simulink model "KR6_Decentralized_Trajectory"  (R2018a)
settings: Solver=VariableStepAuto  StartTime=0.0  StopTime=20  RelTol=1e-3
values from neighbouring files (symbols this model uses):
  Kd_Decent = zeros(7,7)    [ControlSetup.m]
  Kp_Decent = zeros(7,7)    [ControlSetup.m]
libraries: vrlib x8, KR6_Lib x2, dspinverses x1, realtime_pacer_lib x1
(part 1 of 2)
settings Model: Creator=Pedro Ramalho  LastModifiedBy=Pedro Ramalho
settings DataIOCC: ReturnWorkspaceOutputs=on  ReturnWorkspaceOutputsName=Centralized

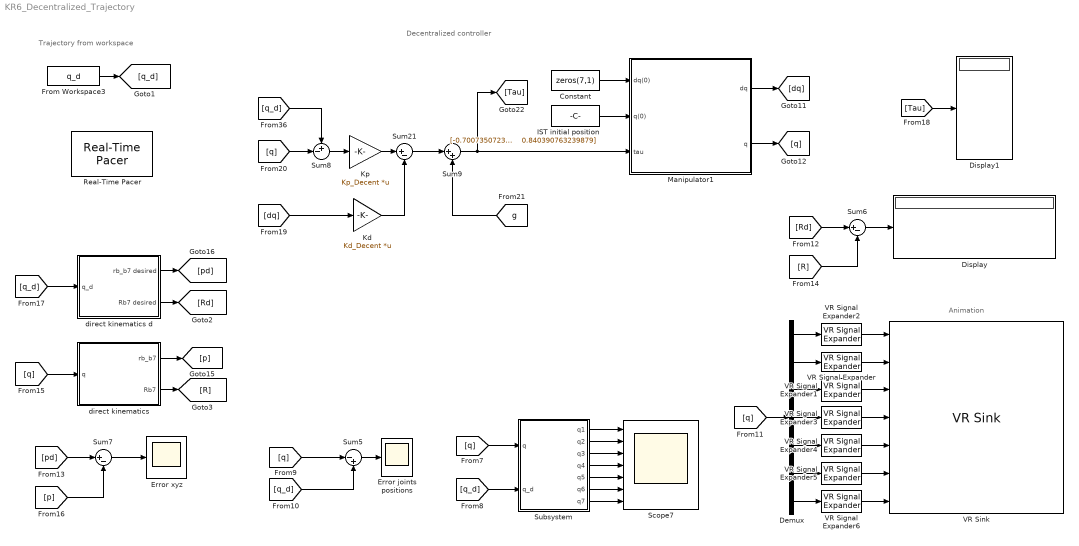
== system KR6_Decentralized_Trajectory ==
  note: Animation
  note: Trajectory from workspace
  note: Decentralized controller
  Constant : Constant  Value=zeros(7,1)
  Demux : Demux  Outputs=7
  Display : Display
  Display1 : Display
  Error joints positions : Scope
  Error xyz : Scope
  From Workspace3 : FromWorkspace  VariableName=q_d  SampleTime=0
  IST initial position : Constant  Value="[-0.700735072364346    0.260226322165590    -1.41409718169695    0.123044715609812    0.767247092108692    -0.379724450954367    0.840390763239879]"
  Kd : Gain  Gain=Kd_Decent  Multiplication=Matrix(K*u)
  Kp : Gain  Gain=Kp_Decent  Multiplication=Matrix(K*u)
  Manipulator1 : Subsystem
  Real-Time Pacer : realtime_pacer_lib/Real-Time Pacer  simTimePerRealTime=1
  Scope7 : Scope  NumInputPorts=7
  Subsystem : Subsystem
  Sum21 : Sum  Inputs=|+-
  Sum5 : Sum  Inputs=|-+
  Sum6 : Sum  Inputs=|+-
  Sum7 : Sum  Inputs=|+-
  Sum8 : Sum  Inputs=+-|
  Sum9 : Sum  Inputs=|++
  VR Signal Expander{,1,3..6} (6 alike) : vrlib/VR Signal Expander  outwidth=4  outidx=4
      settings: SourceProductName=Simulink 3D Animation  SourceProductBaseCode=VR
  VR Signal Expander2 : vrlib/VR Signal Expander  outwidth=3  outidx=3
      settings: SourceProductName=Simulink 3D Animation  SourceProductBaseCode=VR
  VR Sink : vrlib/VR Sink  InstantiateOnLoad=on  SampleTime=0.1  ViewEnable=on  RemoteChange=off  RemoteView=off  FieldsWritten=Jt1_DH_dv.translation.3.1.1.double#Jt2_DH_dv.rotation.4.1.1.double#Jt3_DH_dv.rotation.4.1.1.double#Jt4_DH_dv.rotation.4.1.1.double#Jt5_DH_dv.rotation.4.1.1.double#Jt6_DH_dv.rotation.4.1.1.double#Jt7_DH_dv.rotation.4.1.1.double  WorldFileName=vrrobotKR6.wrl  WorldDescription=D-H Reference Frames for Virtual Reality Robot  AutoView=off  VideoDimensions=[]  AllowVariableSize=off
      settings: SourceProductBaseCode=VR
  direct kinematics : Subsystem
  "direct kinematics d " : Subsystem
  wires:
  [q] -> Sum5/1
  [q_d] -> Sum5/2
  Sum5/1 -> Error joints positions/1
  [q] -> Subsystem/1(q)
  [q_d] -> Subsystem/2(q_d)
  Subsystem/1(q1) -> Scope7/1
  Subsystem/2(q2) -> Scope7/2
  Subsystem/3(q3) -> Scope7/3
  Subsystem/4(q4) -> Scope7/4
  Subsystem/5(q5) -> Scope7/5
  Subsystem/6(q6) -> Scope7/6
  Subsystem/7(q7) -> Scope7/7
  Sum7/1 -> Error xyz/1
  [pd] -> Sum7/1
  [p] -> Sum7/2
  [q_d] -> "direct kinematics d "/1(q_d)
  Demux/1 -> VR Signal Expander2/1
  Demux/2 -> VR Signal Expander/1
  VR Signal Expander2/1 -> VR Sink/1
  VR Signal Expander4/1 -> VR Sink/5
  VR Signal Expander/1 -> VR Sink/2
  "direct kinematics d "/1(rb_b7 desired) -> [pd]
  direct kinematics/1("rb_b7 ") -> [p]
  Demux/5 -> VR Signal Expander4/1
  [q] -> direct kinematics/1(q)
  VR Signal Expander5/1 -> VR Sink/6
  Demux/7 -> VR Signal Expander6/1
  VR Signal Expander6/1 -> VR Sink/7
  VR Signal Expander3/1 -> VR Sink/4
  Demux/6 -> VR Signal Expander5/1
  Demux/4 -> VR Signal Expander3/1
  VR Signal Expander1/1 -> VR Sink/3
  Demux/3 -> VR Signal Expander1/1
  From Workspace3/1 -> [q_d]
  [q] -> Demux/1
  "direct kinematics d "/2(Rb7 desired) -> [Rd]
  direct kinematics/2(Rb7) -> [R]
  [R] -> Sum6/2
  Sum6/1 -> Display/1
  [Rd] -> Sum6/1
  [Tau] -> Display1/1
  [q_d] -> Sum8/1
  Sum21/1 -> Sum9/1
  Kp/1 -> Sum21/1
  Sum9/1 -> [Tau], Manipulator1/3(tau)
  Sum8/1 -> Kp/1
  [q] -> Sum8/2
  [dq] -> Kd/1
  [g] -> Sum9/2
  Manipulator1/1(dq) -> [dq]
  Constant/1 -> Manipulator1/1("dq(0) ")
  IST initial position/1 -> Manipulator1/2("q(0) ")
  Kd/1 -> Sum21/2
  Manipulator1/2(q) -> [q]

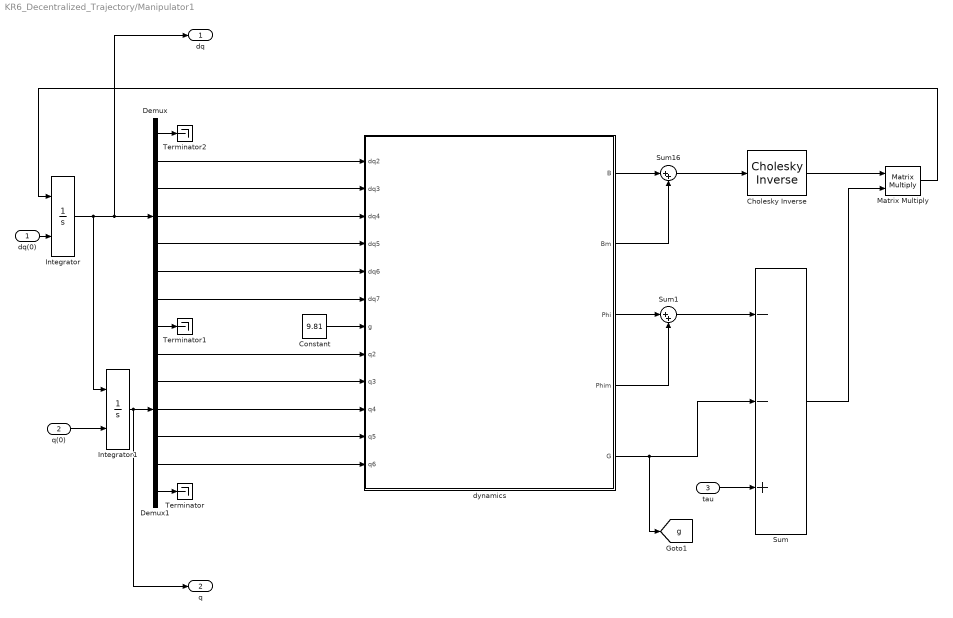
== system KR6_Decentralized_Trajectory/Manipulator1 ==
  "dq(0) " : Inport
  "q(0) " : Inport  Port=2
  tau : Inport  Port=3
  Cholesky Inverse : dspinverses/Cholesky Inverse  errmode=Warning
      settings: SourceProductName=DSP System Toolbox  SourceProductBaseCode=DS
  Constant : Constant  Value=9.81
  Demux : Demux  Outputs=7
  Demux1 : Demux  Outputs=7
  Integrator : Integrator  InitialConditionSource=external
  Integrator1 : Integrator  InitialConditionSource=external
  Matrix Multiply : Product  Multiplication=Matrix(*)
  Sum : Sum  Inputs=--+
  Sum1 : Sum  Inputs=|++
  Sum16 : Sum  Inputs=|++
  Terminator : Terminator
  Terminator1 : Terminator
  Terminator2 : Terminator
  dynamics : MATLAB Function  TreatAsAtomicUnit=on
  dq : Outport
  q : Outport  Port=2
  tag scope: g=global
  wires:
  Sum1/1 -> Sum/1
  Cholesky Inverse/1 -> Matrix Multiply/1
  dynamics/4(Phim) -> Sum1/2
  dynamics/5(G) -> [g], Sum/2
  Integrator/1 -> dq/1, Demux/1, Integrator1/1
  dynamics/1(B) -> Sum16/1
  "dq(0) "/1 -> Integrator/2
  dynamics/2(Bm) -> Sum16/2
  Sum/1 -> Matrix Multiply/2
  Demux1/5 -> dynamics/11(q5)
  Sum16/1 -> Cholesky Inverse/1
  "q(0) "/1 -> Integrator1/2
  dynamics/3(Phi) -> Sum1/1
  Demux1/1 -> Terminator1/1
  Integrator1/1 -> q/1, Demux1/1
  Demux/6 -> dynamics/5(dq6)
  Demux1/4 -> dynamics/10(q4)
  Constant/1 -> dynamics/7(g)
  Demux/2 -> dynamics/1(dq2)
  Demux/3 -> dynamics/2(dq3)
  Demux/4 -> dynamics/3(dq4)
  Demux/5 -> dynamics/4(dq5)
  Demux/7 -> dynamics/6(dq7)
  Matrix Multiply/1 -> Integrator/1
  tau/1 -> Sum/3
  Demux1/6 -> dynamics/12(q6)
  Demux1/2 -> dynamics/8(q2)
  Demux/1 -> Terminator2/1
  Demux1/3 -> dynamics/9(q3)
  Demux1/7 -> Terminator/1

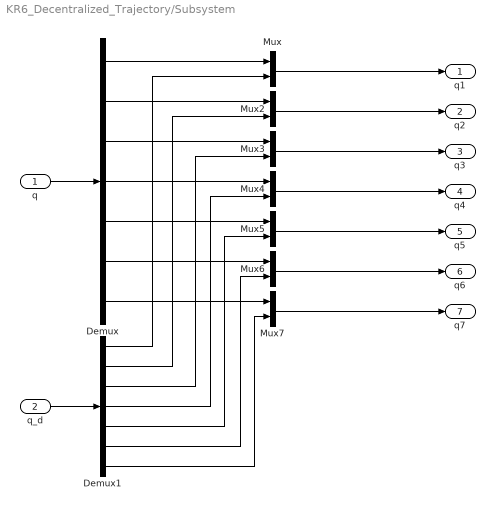
== system KR6_Decentralized_Trajectory/Subsystem ==
  q : Inport
  q_d : Inport  Port=2
  Demux : Demux  Outputs=7
  Demux1 : Demux  Outputs=7
  Mux{,2..7} (7 alike) : Mux  Inputs=2
  q1 : Outport
  q2 : Outport  Port=2
  q3 : Outport  Port=3
  q4 : Outport  Port=4
  q5 : Outport  Port=5
  q6 : Outport  Port=6
  q7 : Outport  Port=7
  wires:
  Demux/3 -> Mux3/1
  Demux/7 -> Mux7/1
  Demux1/6 -> Mux6/2
  Demux1/1 -> Mux/2
  Demux/4 -> Mux4/1
  Demux1/4 -> Mux4/2
  Demux/1 -> Mux/1
  Demux1/5 -> Mux5/2
  Mux4/1 -> q4/1
  Demux1/3 -> Mux3/2
  Demux/2 -> Mux2/1
  Demux1/7 -> Mux7/2
  Demux1/2 -> Mux2/2
  Demux/5 -> Mux5/1
  Demux/6 -> Mux6/1
  Mux6/1 -> q6/1
  q/1 -> Demux/1
  Mux/1 -> q1/1
  Mux3/1 -> q3/1
  Mux2/1 -> q2/1
  Mux5/1 -> q5/1
  Mux7/1 -> q7/1
  q_d/1 -> Demux1/1

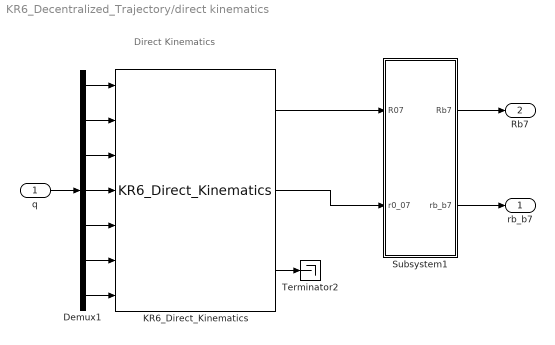
== system KR6_Decentralized_Trajectory/direct kinematics ==
  note: Direct Kinematics
  q : Inport
  Demux1 : Demux  Outputs=7
  KR6_Direct_Kinematics : KR6_Lib/KR6_Direct_Kinematics
  Subsystem1 : Subsystem
  Terminator2 : Terminator
  "rb_b7 " : Outport
  Rb7 : Outport  Port=2
  wires:
  KR6_Direct_Kinematics/3 -> Terminator2/1
  Demux1/1 -> KR6_Direct_Kinematics/1
  Demux1/6 -> KR6_Direct_Kinematics/6
  Demux1/5 -> KR6_Direct_Kinematics/5
  Demux1/3 -> KR6_Direct_Kinematics/3
  KR6_Direct_Kinematics/1 -> Subsystem1/1(R07)
  Subsystem1/1(Rb7) -> Rb7/1
  KR6_Direct_Kinematics/2 -> Subsystem1/2(r0_07)
  Demux1/7 -> KR6_Direct_Kinematics/7
  Demux1/2 -> KR6_Direct_Kinematics/2
  Demux1/4 -> KR6_Direct_Kinematics/4
  q/1 -> Demux1/1
  Subsystem1/2(rb_b7) -> "rb_b7 "/1

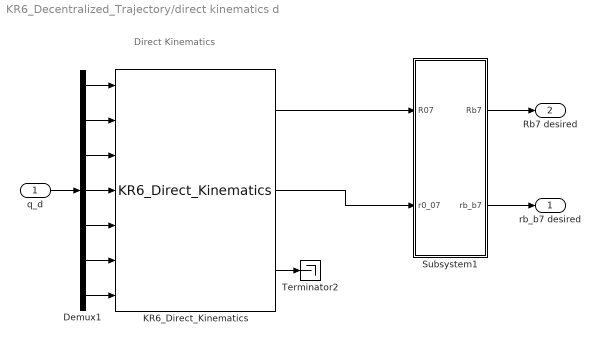
== system KR6_Decentralized_Trajectory/direct kinematics d  ==
  note: Direct Kinematics
  q_d : Inport
  Demux1 : Demux  Outputs=7
  KR6_Direct_Kinematics : KR6_Lib/KR6_Direct_Kinematics
  Subsystem1 : Subsystem
  Terminator2 : Terminator
  rb_b7 desired : Outport
  Rb7 desired : Outport  Port=2
  wires:
  KR6_Direct_Kinematics/1 -> Subsystem1/1(R07)
  KR6_Direct_Kinematics/3 -> Terminator2/1
  Demux1/1 -> KR6_Direct_Kinematics/1
  Demux1/6 -> KR6_Direct_Kinematics/6
  Demux1/5 -> KR6_Direct_Kinematics/5
  Demux1/3 -> KR6_Direct_Kinematics/3
  Subsystem1/1(Rb7) -> Rb7 desired/1
  KR6_Direct_Kinematics/2 -> Subsystem1/2(r0_07)
  Demux1/7 -> KR6_Direct_Kinematics/7
  Demux1/2 -> KR6_Direct_Kinematics/2
  Demux1/4 -> KR6_Direct_Kinematics/4
  q_d/1 -> Demux1/1
  Subsystem1/2(rb_b7) -> rb_b7 desired/1

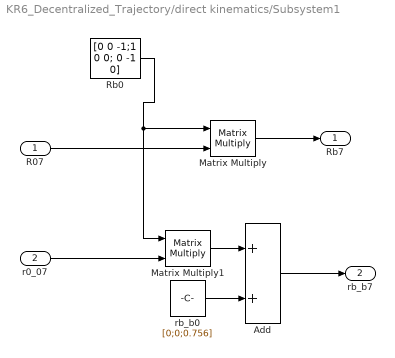
== system KR6_Decentralized_Trajectory/direct kinematics/Subsystem1 ==
  R07 : Inport
  r0_07 : Inport  Port=2
  Add : Sum
  Matrix Multiply : Product  Multiplication=Matrix(*)
  Matrix Multiply1 : Product  Multiplication=Matrix(*)
  Rb0 : Constant  Value=[0 0 -1;1 0 0; 0 -1 0]
  rb_b0 : Constant  Value=[0;0;0.756]
  Rb7 : Outport
  rb_b7 : Outport  Port=2
  wires:
  R07/1 -> Matrix Multiply/2
  r0_07/1 -> Matrix Multiply1/2
  Matrix Multiply/1 -> Rb7/1
  Rb0/1 -> Matrix Multiply1/1, Matrix Multiply/1
  Matrix Multiply1/1 -> Add/1
  rb_b0/1 -> Add/2
  Add/1 -> rb_b7/1

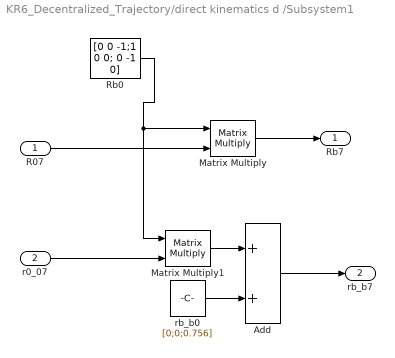
== system KR6_Decentralized_Trajectory/direct kinematics d /Subsystem1 ==
  R07 : Inport
  r0_07 : Inport  Port=2
  Add : Sum
  Matrix Multiply : Product  Multiplication=Matrix(*)
  Matrix Multiply1 : Product  Multiplication=Matrix(*)
  Rb0 : Constant  Value=[0 0 -1;1 0 0; 0 -1 0]
  rb_b0 : Constant  Value=[0;0;0.756]
  Rb7 : Outport
  rb_b7 : Outport  Port=2
  wires:
  R07/1 -> Matrix Multiply/2
  r0_07/1 -> Matrix Multiply1/2
  Matrix Multiply/1 -> Rb7/1
  Rb0/1 -> Matrix Multiply1/1, Matrix Multiply/1
  Matrix Multiply1/1 -> Add/1
  rb_b0/1 -> Add/2
  Add/1 -> rb_b7/1
